simulink model "control"  (R2023b)
settings: Solver=VariableStepAuto  StartTime=0.0  StopTime=10.0  RelTol=1e-3
libraries: robotcorelib x2
settings Model: Creator=jake9  LastModifiedBy=jake9

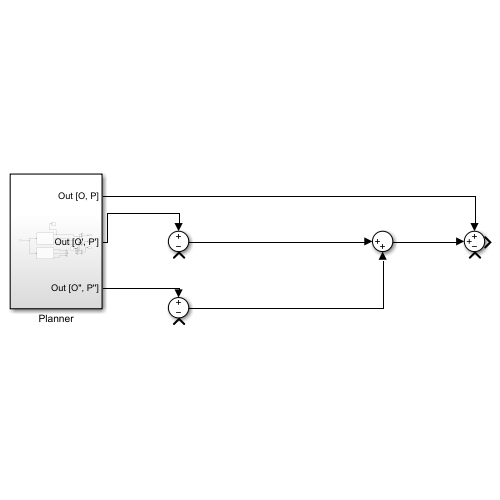
[thumbnail: Simulink's stored preview of the top-level diagram]
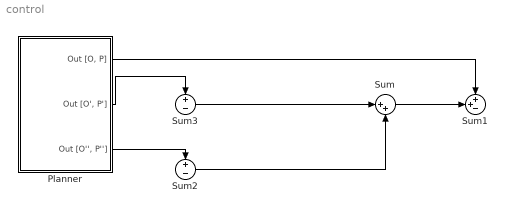
== system control ==
  Planner : Subsystem
  Sum : Sum  Inputs=|++
  Sum1 : Sum  Inputs=++-
  Sum2 : Sum  Inputs=+-
  Sum3 : Sum  Inputs=+-
  wires:
  Planner/1("Out [O, P]") -> Sum1/1
  Planner/2("Out [O', P']") -> Sum3/1
  Planner/3("Out [O'', P'']") -> Sum2/1
  Sum3/1 -> Sum/1
  Sum2/1 -> Sum/2
  Sum/1 -> Sum1/2

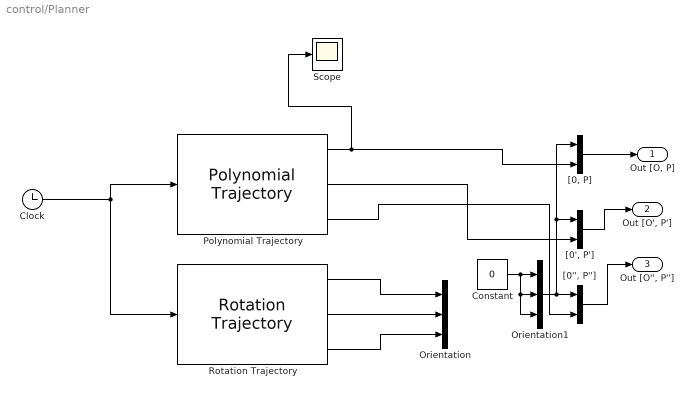
== system control/Planner ==
  Clock : Clock
  Constant : Constant  Value=0
  Orientation : Mux  Inputs=3
  Orientation1 : Mux  Inputs=3
  Polynomial Trajectory : robotcorelib/Polynomial Trajectory  WaypointSource=Internal  Waypoints=[1 1 1; 2 2 2; 3 3 3]'  TimePoints=[0, 4, 8]  TimeInterval=[ 1, 4 ]  Method=Cubic Polynomial  ParameterSource=Internal  VelocityBoundaryCondition=zeros( 3,3 )  AccelerationBoundaryCondition=zeros( 2, 5 )  SimulateUsing=Interpreted execution
  Rotation Trajectory : robotcorelib/Rotation Trajectory  WaypointFormat=Quaternion  WaypointSource=Internal  R0=[ 1, 0, 0, 0 ]'  RF=[ 0, 0, 1, 0 ]'  TimeInterval=[ 0, 8]  CustomTimeScaling=off  ParameterSource=Internal  TSTime=0:0.1:1  TimeScaling=[ 0:0.1:1; ones( 1, 11 ); zeros( 1, 11 ) ]  SimulateUsing=Interpreted execution
      settings: LibrarySourceBlock=robotutilslib/Rotation Trajectory
  Scope : Scope
  "[0'', P'']" : Mux  Inputs=2
  "[0', P']" : Mux  Inputs=2
  "[0, P]" : Mux  Inputs=2
  "Out [O, P]" : Outport
  "Out [O', P']" : Outport  Port=2
  "Out [O'', P'']" : Outport  Port=3
  wires:
  Clock/1 -> Rotation Trajectory/1, Polynomial Trajectory/1
  Polynomial Trajectory/1 -> "[0, P]"/2, Scope/1
  Polynomial Trajectory/2 -> "[0', P']"/2
  Polynomial Trajectory/3 -> "[0'', P'']"/2
  Rotation Trajectory/3 -> Orientation/3
  Rotation Trajectory/2 -> Orientation/2
  Rotation Trajectory/1 -> Orientation/1
  "[0, P]"/1 -> "Out [O, P]"/1
  Constant/1 -> Orientation1/3, Orientation1/2, Orientation1/1
  Orientation1/1 -> "[0'', P'']"/1, "[0', P']"/1, "[0, P]"/1
  "[0', P']"/1 -> "Out [O', P']"/1
  "[0'', P'']"/1 -> "Out [O'', P'']"/1
